simulink model "lookup_nD_TestGen32"  (R2017b)
settings: Solver=FixedStepDiscrete  StartTime=0.0  StopTime=10.0  RelTol=1e-3
undefined symbols (not defined in the file): Block_TestLib, enable_trigger
settings Model: Creator=ktrinh  LastModifiedBy=ktrinh
settings DebuggingCC: ParameterOverflowMsg=none

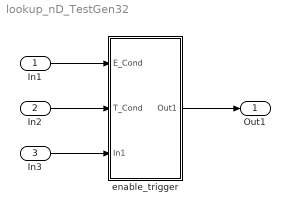
== system lookup_nD_TestGen32 ==
  In1 : Inport
  In2 : Inport  Port=2
  In3 : Inport  Port=3
  enable_trigger : Subsystem  AncestorBlock=Block_TestLib/enable_trigger
  Out1 : Outport
  wires:
  In1/1 -> enable_trigger/1(E_Cond)
  In2/1 -> enable_trigger/2(T_Cond)
  In3/1 -> enable_trigger/3(In1)
  enable_trigger/1(Out1) -> Out1/1

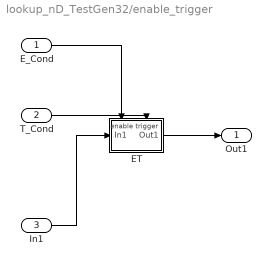
== system lookup_nD_TestGen32/enable_trigger ==
  E_Cond : Inport  OutDataTypeStr=boolean
  T_Cond : Inport  Port=2  OutDataTypeStr=boolean
  In1 : Inport  Port=3
  ET : Subsystem  TreatAsAtomicUnit=on
  Out1 : Outport
  wires:
  T_Cond/1 -> ET/Trigger
  E_Cond/1 -> ET/Enable
  In1/1 -> ET/1(In1)
  ET/1(Out1) -> Out1/1

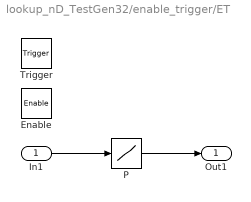
== system lookup_nD_TestGen32/enable_trigger/ET ==
  In1 : Inport  PortDimensions=6
  Enable : EnablePort
  Trigger : TriggerPort  VariantControl=Variant
  P : Lookup_n-D  NumberOfTableDimensions=6  BreakpointsSpecification=Even spacing  BreakpointsForDimension3=[5, 7]  BreakpointsForDimension1FirstPoint=80.9114  BreakpointsForDimension2FirstPoint=16.6565  BreakpointsForDimension3FirstPoint=114.6232  BreakpointsForDimension4FirstPoint=116.7491  BreakpointsForDimension5FirstPoint=70.5143  BreakpointsForDimension6FirstPoint=41.5036  BreakpointsForDimension1Spacing=1.5  BreakpointsForDimension2Spacing=1.5  BreakpointsForDimension3Spacing=1.5  BreakpointsForDimension4Spacing=1.5  BreakpointsForDimension5Spacing=1.5  BreakpointsForDimension6Spacing=1.5  UseOneInputPortForAllInputData=on  Table=reshape(repmat([4 5 6 7 8;16 19 20 21 22;10 18 23 24 25],6,8),[2,5,3,2,3, 4])  InterpMethod=Flat  UseLastTableValue=on  InternalRulePriority=Speed  RndMeth=Simplest  InputSameDT=on
  Out1 : Outport
  wires:
  In1/1 -> P/1
  P/1 -> Out1/1
